simulink model "PID_controller_v02"  (R2019a)
settings: Solver=VariableStepAuto  StartTime=0.0  StopTime=10  FixedStep=0.001  RelTol=1e-4
values from neighbouring files (symbols this model uses):
  den = cell2mat(H(1).Denominator)    [control_system_v01.m]    (also in control_system_v02.m = H.Denominator)
  num = cell2mat(H(1).Numerator)    [control_system_v01.m]    (also in control_system_v02.m = H.Numerator)
libraries: simulink x3
settings Model: Creator=tyson  LastModifiedBy=tyson

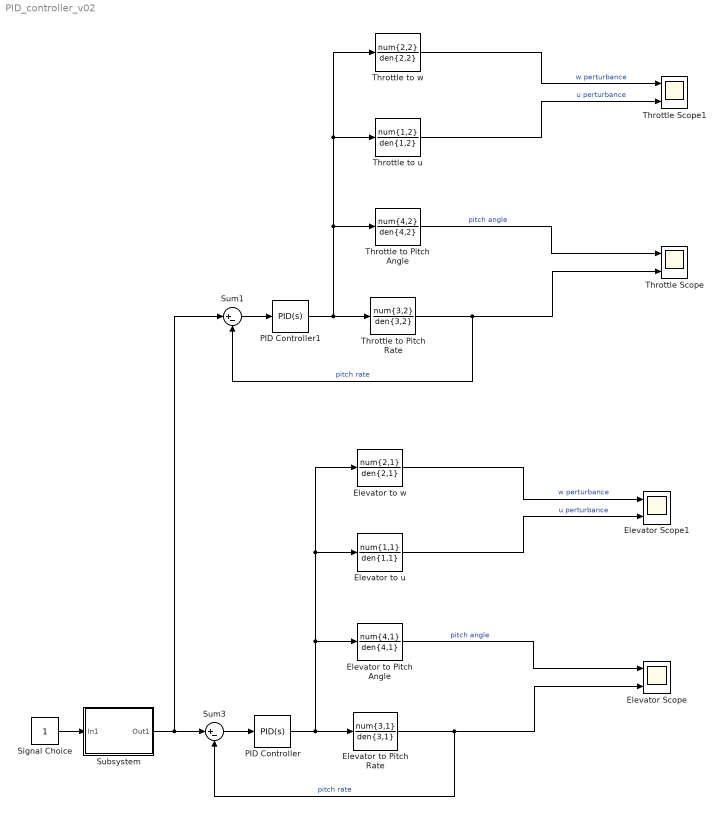
== system PID_controller_v02 ==
  Elevator Scope : Scope  NumInputPorts=2
  Elevator Scope1 : Scope  NumInputPorts=2
  Elevator to Pitch Angle : TransferFcn  Numerator=num{4,1}  Denominator=den{4,1}
  Elevator to Pitch Rate : TransferFcn  Numerator=num{3,1}  Denominator=den{3,1}
  Elevator to u : TransferFcn  Numerator=num{1,1}  Denominator=den{1,1}
  Elevator to w : TransferFcn  Numerator=num{2,1}  Denominator=den{2,1}
  PID Controller : simulink/Continuous/PID Controller  Controller=PID  Form=Parallel  TimeDomain=Continuous-time  SampleTime=-1  IntegratorMethod=Forward Euler  FilterMethod=Forward Euler  ControllerParametersSource=internal  P=-1.27272767688815  I=-94.3558471125145  D=5.568325695423e-05  UseFilter=on  N=22856.5595208321  TunerSelectOption=Transfer Function Based (PID Tuner App)  InitialConditionSource=internal  InitialConditionForIntegrator=0  InitialConditionForFilter=0  DifferentiatorICPrevScaledInput=0  ExternalReset=none  TrackingMode=off  Kt=1  LimitOutput=off  UpperSaturationLimit=inf  LowerSaturationLimit=-inf  LinearizeAsGain=on  AntiWindupMode=none  Kb=1  POutMin=[]  POutMax=[]  IOutMin=[]  IOutMax=[]  DOutMin=[]  DOutMax=[]  NOutMin=[]  NOutMax=[]  SumOutMin=[]  SumOutMax=[]  SaturationOutMin=[]  SaturationOutMax=[]  PParamMin=[]  PParamMax=[]  IParamMin=[]  IParamMax=[]  DParamMin=[]  DParamMax=[]  NParamMin=[]  NParamMax=[]  KbParamMin=[]  KbParamMax=[]  KtParamMin=[]  KtParamMax=[]  KbOutMin=[]  KbOutMax=[]  KtOutMin=[]  KtOutMax=[]  IntegratorOutMin=[]  IntegratorOutMax=[]  FilterOutMin=[]  FilterOutMax=[]  SumI1OutMin=[]  SumI1OutMax=[]  SumI2OutMin=[]  SumI2OutMax=[]  SumI3OutMin=[]  SumI3OutMax=[]  SumI4OutMin=[]  SumI4OutMax=[]  SumDOutMin=[]  SumDOutMax=[]  DifferentiatorOutMin=[]  DifferentiatorOutMax=[]  FilterDiffOutCoefMin=[]  FilterDiffOutCoefMax=[]  ReciprocalOutMin=[]  ReciprocalOutMax=[]  SumDenOutMin=[]  SumDenOutMax=[]  SumNumOutMin=[]  SumNumOutMax=[]  DivideOutMin=[]  DivideOutMax=[]  IntegratorContinuousStateAttributes=''  IntegratorStateMustResolveToSignalObject=off  IntegratorRTWStateStorageClass=Auto  FilterContinuousStateAttributes=''  FilterStateMustResolveToSignalObject=off  FilterRTWStateStorageClass=Auto  ParallelPVariant=InternalParameters  IdealPVariant=Disabled  IVariant=InternalParameters  DVariant=InternalParameters  IntegratorVariant=Continuous  SatVariant=Disabled  AWVariant=Passthrough  PCopyVariant=Disabled  TRVariant=Disabled  FdbkBlocksVariant=Forward  IdealPFdbkVariant=Disabled  SatFdbkVariant=Disabled  DerivativeFilterVariant=ContFilter  NVariant=InternalParameters  NCopyVariant=Disabled  FilterICVariant=InternalICsFilter  IntegratorICVariant=InternalICs  ExternalResetVariant=Disabled  TRSumVariant=Passthrough  SumFdbkVariant=Disabled  SumVariant=Sum_PID
  PID Controller1 : simulink/Continuous/PID Controller  Controller=PID  Form=Parallel  TimeDomain=Continuous-time  SampleTime=-1  IntegratorMethod=Forward Euler  FilterMethod=Forward Euler  ControllerParametersSource=internal  P=5.37331737198142  I=12.5200222602471  D=0.218316613438136  UseFilter=on  N=1624.62758050326  TunerSelectOption=Transfer Function Based (PID Tuner App)  InitialConditionSource=internal  InitialConditionForIntegrator=0  InitialConditionForFilter=0  DifferentiatorICPrevScaledInput=0  ExternalReset=none  TrackingMode=off  Kt=1  LimitOutput=off  UpperSaturationLimit=inf  LowerSaturationLimit=-inf  LinearizeAsGain=on  AntiWindupMode=none  Kb=1  POutMin=[]  POutMax=[]  IOutMin=[]  IOutMax=[]  DOutMin=[]  DOutMax=[]  NOutMin=[]  NOutMax=[]  SumOutMin=[]  SumOutMax=[]  SaturationOutMin=[]  SaturationOutMax=[]  PParamMin=[]  PParamMax=[]  IParamMin=[]  IParamMax=[]  DParamMin=[]  DParamMax=[]  NParamMin=[]  NParamMax=[]  KbParamMin=[]  KbParamMax=[]  KtParamMin=[]  KtParamMax=[]  KbOutMin=[]  KbOutMax=[]  KtOutMin=[]  KtOutMax=[]  IntegratorOutMin=[]  IntegratorOutMax=[]  FilterOutMin=[]  FilterOutMax=[]  SumI1OutMin=[]  SumI1OutMax=[]  SumI2OutMin=[]  SumI2OutMax=[]  SumI3OutMin=[]  SumI3OutMax=[]  SumI4OutMin=[]  SumI4OutMax=[]  SumDOutMin=[]  SumDOutMax=[]  DifferentiatorOutMin=[]  DifferentiatorOutMax=[]  FilterDiffOutCoefMin=[]  FilterDiffOutCoefMax=[]  ReciprocalOutMin=[]  ReciprocalOutMax=[]  SumDenOutMin=[]  SumDenOutMax=[]  SumNumOutMin=[]  SumNumOutMax=[]  DivideOutMin=[]  DivideOutMax=[]  IntegratorContinuousStateAttributes=''  IntegratorStateMustResolveToSignalObject=off  IntegratorRTWStateStorageClass=Auto  FilterContinuousStateAttributes=''  FilterStateMustResolveToSignalObject=off  FilterRTWStateStorageClass=Auto  ParallelPVariant=InternalParameters  IdealPVariant=Disabled  IVariant=InternalParameters  DVariant=InternalParameters  IntegratorVariant=Continuous  SatVariant=Disabled  AWVariant=Passthrough  PCopyVariant=Disabled  TRVariant=Disabled  FdbkBlocksVariant=Forward  IdealPFdbkVariant=Disabled  SatFdbkVariant=Disabled  DerivativeFilterVariant=ContFilter  NVariant=InternalParameters  NCopyVariant=Disabled  FilterICVariant=InternalICsFilter  IntegratorICVariant=InternalICs  ExternalResetVariant=Disabled  TRSumVariant=Passthrough  SumFdbkVariant=Disabled  SumVariant=Sum_PID
  Signal Choice : Constant
  Subsystem : Subsystem  Description=Input Signal
  Sum1 : Sum  Inputs=|+-
  Sum3 : Sum  Inputs=|+-
  Throttle Scope : Scope  NumInputPorts=2
  Throttle Scope1 : Scope  NumInputPorts=2
  Throttle to Pitch Angle : TransferFcn  Numerator=num{4,2}  Denominator=den{4,2}
  Throttle to Pitch Rate : TransferFcn  Numerator=num{3,2}  Denominator=den{3,2}
  Throttle to u : TransferFcn  Numerator=num{1,2}  Denominator=den{1,2}
  Throttle to w : TransferFcn  Numerator=num{2,2}  Denominator=den{2,2}
  wires:
  Elevator to Pitch Rate/1 -> Sum3/2, Elevator Scope/2  "pitch rate"
  PID Controller/1 -> Elevator to w/1, Elevator to u/1, Elevator to Pitch Angle/1, Elevator to Pitch Rate/1
  Sum3/1 -> PID Controller/1
  Elevator to u/1 -> Elevator Scope1/2  "u perturbance"
  Elevator to w/1 -> Elevator Scope1/1  "w perturbance"
  Elevator to Pitch Angle/1 -> Elevator Scope/1  "pitch angle"
  Signal Choice/1 -> Subsystem/1(In1)
  Throttle to Pitch Angle/1 -> Throttle Scope/1  "pitch angle"
  Throttle to w/1 -> Throttle Scope1/1  "w perturbance"
  Subsystem/1(Out1) -> Sum1/1, Sum3/1
  Throttle to Pitch Rate/1 -> Sum1/2, Throttle Scope/2  "pitch rate"
  Throttle to u/1 -> Throttle Scope1/2  "u perturbance"
  Sum1/1 -> PID Controller1/1
  PID Controller1/1 -> Throttle to w/1, Throttle to u/1, Throttle to Pitch Angle/1, Throttle to Pitch Rate/1

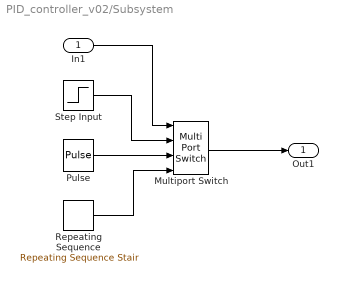
== system PID_controller_v02/Subsystem ==
  In1 : Inport
  Multiport Switch : MultiPortSwitch  InputSameDT=on
  "Pulse " : DiscretePulseGenerator  PulseType=Time based  Period=5  PulseWidth=20
  "Repeating Sequence " : simulink/Sources/Repeating Sequence Stair  OutValues=[1 1 1 1 1 0 0 0 0 0 -1 -1 -1 -1 -1 0 0 0 0 0].'  tsamp=-1  OutMin=[]  OutMax=[]  OutDataTypeStr=double  OutputDataTypeScalingMode=double  OutDataType=fixdt(0,8)  ConRadixGroup=Best Precision: Vector-wise  OutScaling=2^-12
  Step Input : Step  Time=0
  Out1 : Outport
  wires:
  Multiport Switch/1 -> Out1/1
  "Pulse "/1 -> Multiport Switch/3
  Step Input/1 -> Multiport Switch/2
  In1/1 -> Multiport Switch/1
  "Repeating Sequence "/1 -> Multiport Switch/4
